simulink model "squaredExponentialCovMat_ts"  (R2018b)
settings: Solver=VariableStepAuto  StartTime=0.0  StopTime=0  RelTol=1e-3
values from neighbouring files (symbols this model uses):
  covarianceAmp = 0.05    [buildCovarianceMatrix_ta.m]
  dsgnSet1 = rand(2,8)    [buildCovarianceMatrix_ta.m]
  dsgnSet2 = rand(2,1)    [buildCovarianceMatrix_ta.m]
  lengthScale = [1;1]    [buildCovarianceMatrix_ta.m]
  noiseVariance = 0.1    [buildCovarianceMatrix_ta.m]
libraries: buildSqrdExpCovMat x1
settings Model: Creator=Ayaz  LastModifiedBy=asiddiq2

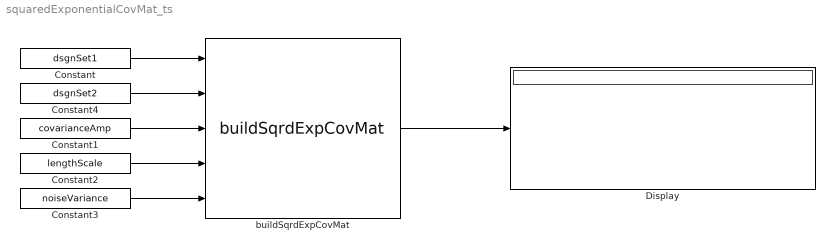
== system squaredExponentialCovMat_ts ==
  Constant : Constant  Value=dsgnSet1  VectorParams1D=off
  Constant1 : Constant  Value=covarianceAmp  VectorParams1D=off
  Constant2 : Constant  Value=lengthScale  VectorParams1D=off
  Constant3 : Constant  Value=noiseVariance  VectorParams1D=off
  Constant4 : Constant  Value=dsgnSet2  VectorParams1D=off
  Display : Display
  buildSqrdExpCovMat : buildSqrdExpCovMat/buildSqrdExpCovMat  SystemSampleTime=-1
  wires:
  buildSqrdExpCovMat/1 -> Display/1
  Constant1/1 -> buildSqrdExpCovMat/3
  Constant4/1 -> buildSqrdExpCovMat/2
  Constant2/1 -> buildSqrdExpCovMat/4
  Constant/1 -> buildSqrdExpCovMat/1
  Constant3/1 -> buildSqrdExpCovMat/5
